simulink model "feedbackonly"  (Simulink 7.4)
settings: Solver=ode45  StartTime=0.0  StopTime=15  FixedStep=0.01  RelTol=1e-3
values from neighbouring files (symbols this model uses):
  A = [((-(Km^2)/(Rm*Jt))-(bs/Jt)) 0 0 0 ... (first row only)    [tilstandsREG.m]
  B = [1.292*(Km/(Jt*Rm)) ... (first row only)    [tilstandsREG.m]
  C = [1 0 0 0 ... (first row only)    [tilstandsREG.m]
  F = Fe(:,1:4)    [tilstandsREG.m]
settings Model: Creator=Skov  LastModifiedBy=Skov

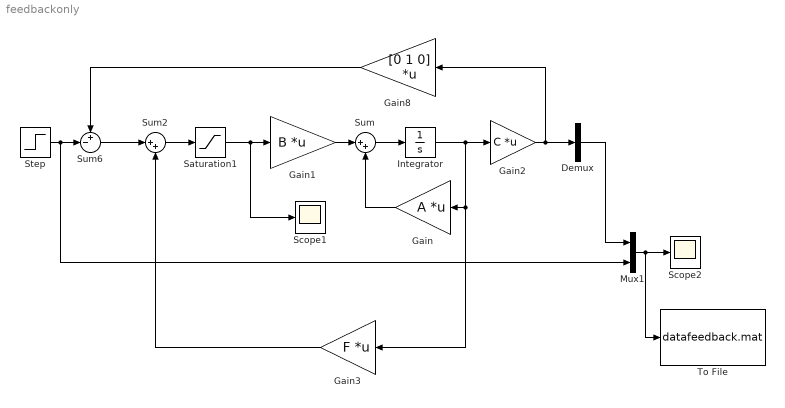
== system feedbackonly ==
  Demux : Demux  Outputs=3
  Gain : Gain  Gain=A  Multiplication=Matrix(K*u)  ParameterDataType=fixdt(1, 16)  ParameterScaling=2^0  OutDataType=fixdt(1, 16)  OutScaling=2^0
  Gain1 : Gain  Gain=B  Multiplication=Matrix(K*u)  ParameterDataType=fixdt(1, 16)  ParameterScaling=2^0  OutDataType=fixdt(1, 16)  OutScaling=2^0
  Gain2 : Gain  Gain=C  Multiplication=Matrix(K*u)  ParameterDataType=fixdt(1, 16)  ParameterScaling=2^0  OutDataType=fixdt(1, 16)  OutScaling=2^0
  Gain3 : Gain  Gain=F  Multiplication=Matrix(K*u)  ParameterDataType=fixdt(1, 16)  ParameterScaling=2^0  OutDataType=fixdt(1, 16)  OutScaling=2^0
  Gain8 : Gain  Gain=[0 1 0]  Multiplication=Matrix(K*u)  ParameterDataType=fixdt(1, 16)  ParameterScaling=2^0  OutDataType=fixdt(1, 16)  OutScaling=2^0
  Integrator : Integrator  InitialCondition=[0 0 0 0]
  Mux1 : Mux  Inputs=2
  Saturation1 : Saturate  UpperLimit=10  LowerLimit=-10  OutDataType=fixdt(1, 16)  OutScaling=2^0
  Scope1 : Scope
      settings: YMin=10  YMax=10
  Scope2 : Scope
      settings: YMin=-0.05  YMax=0.45  SaveName=ScopeData2
  Step : Step  After=pi/6  SampleTime=0
  Sum : Sum  Inputs=|++  OutDataType=fixdt(1, 16)  OutScaling=2^0
  Sum2 : Sum  Inputs=|++  OutDataType=fixdt(1, 16)  OutScaling=2^0
  Sum6 : Sum  Inputs=+-|  OutDataType=fixdt(1, 16)  OutScaling=2^0
  To File : ToFile  Filename=datafeedback.mat
  wires:
  Gain8/1 -> Sum6/1
  Step/1 -> Sum6/2, Mux1/2
  Gain1/1 -> Sum/1
  Integrator/1 -> Gain2/1, Gain/1, Gain3/1
  Sum/1 -> Integrator/1
  Gain/1 -> Sum/2
  Gain2/1 -> Gain8/1, Demux/1
  Mux1/1 -> Scope2/1, To File/1
  Sum6/1 -> Sum2/1
  Gain3/1 -> Sum2/2
  Sum2/1 -> Saturation1/1
  Saturation1/1 -> Gain1/1, Scope1/1
  Demux/2 -> Mux1/1
